simulink model "andgate2"  (R2020a)
settings: Solver=VariableStepAuto  StartTime=0.0  StopTime=inf  RelTol=1e-3
settings Model: Creator=F1  LastModifiedBy=F1

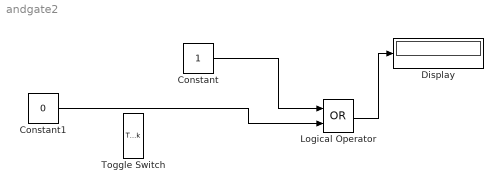
== system andgate2 ==
  Constant : Constant
  Constant1 : Constant  Value=0
  Display : Display
  Logical Operator : Logic  Operator=OR  AllPortsSameDT=off  OutDataTypeStr=boolean
  Toggle Switch : ToggleSwitchBlock
      settings: Values={{'Off', 'On'}, [0 1]}
  wires:
  Constant/1 -> Logical Operator/1
  Logical Operator/1 -> Display/1
  Constant1/1 -> Logical Operator/2
